simulink model "feedback_linearization"  (R2024a)
settings: Solver=VariableStepAuto  StartTime=0.0  StopTime=10.0  RelTol=1e-3
undefined symbols (not defined in the file): k1, k2
settings Model: Creator=ADMIN  LastModifiedBy=ADMIN

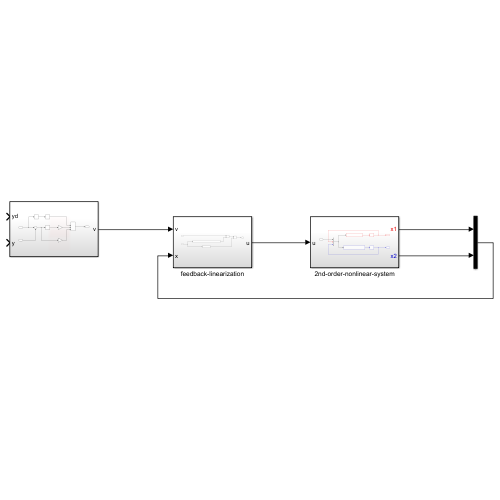
[thumbnail: Simulink's stored preview of the top-level diagram]
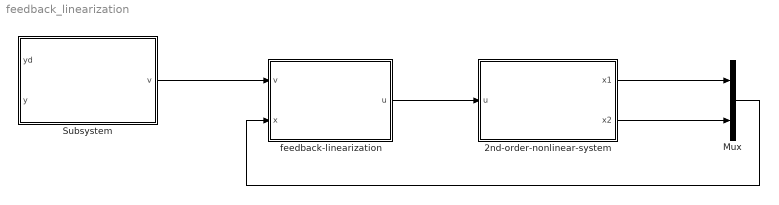
== system feedback_linearization ==
  2nd-order-nonlinear-system : Subsystem
  Mux : Mux  Inputs=2
  Subsystem : Subsystem
  feedback-linearization : Subsystem
  wires:
  feedback-linearization/1(u) -> 2nd-order-nonlinear-system/1(u)
  2nd-order-nonlinear-system/1(x1) -> Mux/1
  2nd-order-nonlinear-system/2(x2) -> Mux/2
  Mux/1 -> feedback-linearization/2(x)
  Subsystem/1(v) -> feedback-linearization/1(v)

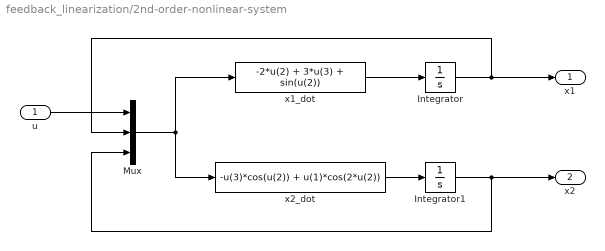
== system feedback_linearization/2nd-order-nonlinear-system ==
  u : Inport
  Integrator : Integrator
  Integrator1 : Integrator
  Mux : Mux  Inputs=3
  x1_dot : Fcn  Expr=-2*u(2) + 3*u(3) + sin(u(2))
  x2_dot : Fcn  Expr=-u(3)*cos(u(2)) + u(1)*cos(2*u(2))
  x1 : Outport
  x2 : Outport  Port=2
  wires:
  x1_dot/1 -> Integrator/1
  Mux/1 -> x2_dot/1, x1_dot/1
  Integrator/1 -> x1/1, Mux/2
  Integrator1/1 -> x2/1, Mux/3
  u/1 -> Mux/1
  x2_dot/1 -> Integrator1/1

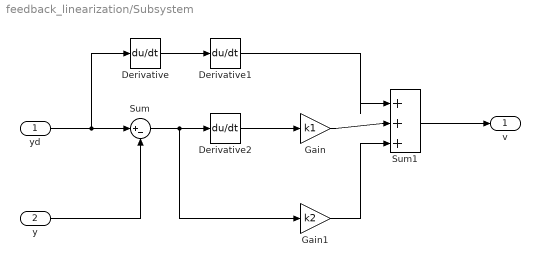
== system feedback_linearization/Subsystem ==
  yd : Inport
  y : Inport  Port=2
  Derivative : Derivative
  Derivative1 : Derivative
  Derivative2 : Derivative
  Gain : Gain  Gain=k1
  Gain1 : Gain  Gain=k2
  Sum : Sum  Inputs=|+-
  Sum1 : Sum  Inputs=|+++
  v : Outport
  wires:
  Gain1/1 -> Sum1/3
  yd/1 -> Sum/1, Derivative/1
  Derivative/1 -> Derivative1/1
  Derivative2/1 -> Gain/1
  y/1 -> Sum/2
  Derivative1/1 -> Sum1/1
  Gain/1 -> Sum1/2
  Sum/1 -> Derivative2/1, Gain1/1
  Sum1/1 -> v/1

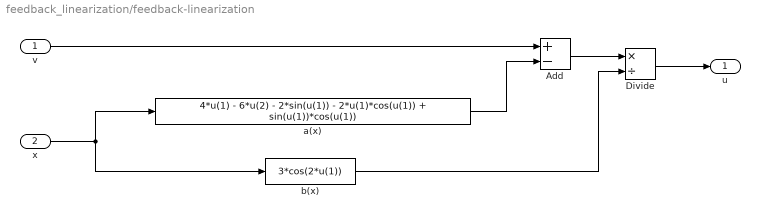
== system feedback_linearization/feedback-linearization ==
  v : Inport
  x : Inport  Port=2
  Add : Sum  Inputs=+-
  Divide : Product  Inputs=*/
  a(x) : Fcn  Expr=4*u(1) - 6*u(2) - 2*sin(u(1)) - 2*u(1)*cos(u(1)) + sin(u(1))*cos(u(1))
  b(x) : Fcn  Expr=3*cos(2*u(1))
  u : Outport
  wires:
  x/1 -> a(x)/1, b(x)/1
  Add/1 -> Divide/1
  v/1 -> Add/1
  Divide/1 -> u/1
  b(x)/1 -> Divide/2
  a(x)/1 -> Add/2
